simulink model "phase"  (R2015b)
settings: Solver=VariableStepAuto  StartTime=0.0  StopTime=10  MaxStep=1e-4  RelTol=1e-3
libraries: simulink x1
settings Model: Creator=yehuohanxing  LastModifiedBy=yehuohanxing

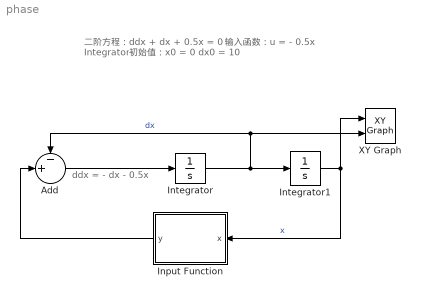
== system phase ==
  note: ddx = - dx - 0.5x
  note: 二阶方程：ddx + dx + 0.5x = 0
      | 输入函数：u = - 0.5x
      | Integrator初始值：x0 = 0
      |                   dx0 = 10
  Add : Sum  Inputs=-+|
  Input Function : MATLAB Function  TreatAsAtomicUnit=on
  Integrator : Integrator  InitialCondition=10
  Integrator1 : Integrator
  XY Graph : simulink/Sinks/XY Graph  xmin=-15  xmax=15  ymin=-15  ymax=15  st=0.1
  wires:
  Integrator/1 -> Integrator1/1, Add/1, XY Graph/2  "dx"
  Add/1 -> Integrator/1
  Integrator1/1 -> Input Function/1(x), XY Graph/1  "x"
  Input Function/1(y) -> Add/2

== matlab function phase/Input Function ==
  data: x input; y output
function y = fcn(x)
y = -0.5*x;
